simulink model "simulate_filter"  (R2023a)
settings: Solver=VariableStepAuto  StartTime=0.0  StopTime=50  RelTol=1e-3
settings Model: Creator=belov  LastModifiedBy=belov

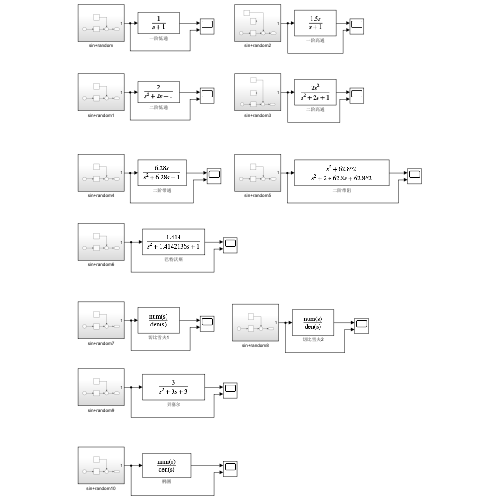
[thumbnail: Simulink's stored preview of the top-level diagram]
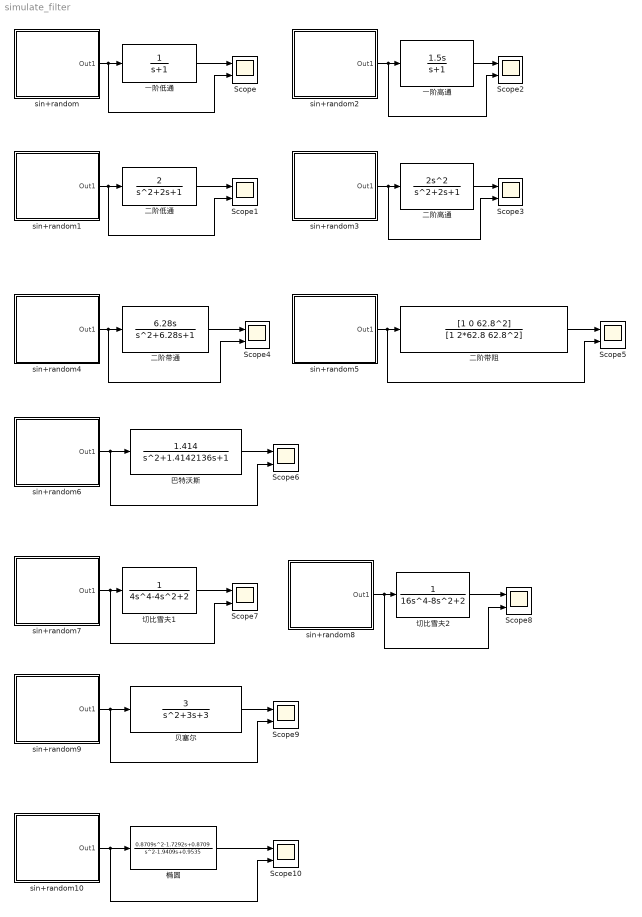
== system simulate_filter ==
  Scope{,1..10} (11 alike) : Scope  NumInputPorts=2
  sin+random : Subsystem
  sin+random1 : Subsystem
  sin+random10 : Subsystem
  sin+random2 : Subsystem
  sin+random3 : Subsystem
  sin+random4 : Subsystem
  sin+random5 : Subsystem
  sin+random6 : Subsystem
  sin+random7 : Subsystem
  sin+random8 : Subsystem
  sin+random9 : Subsystem
  一阶低通 : TransferFcn  Numerator=1  Denominator=[1 1]
  一阶高通 : TransferFcn  Numerator=[1.5 0]  Denominator=[1 1]
  二阶低通 : TransferFcn  Numerator=2
  二阶带通 : TransferFcn  Numerator=[0 6.28 0]  Denominator=[1 6.28 1]
  二阶带阻 : TransferFcn  Numerator=[1 0 62.8^2]  Denominator=[1 2*62.8 62.8^2]
  二阶高通 : TransferFcn  Numerator=[2 0 0]
  切比雪夫1 : TransferFcn  Numerator=1  Denominator=[4 0 -4 0 2]
  切比雪夫2 : TransferFcn  Numerator=1  Denominator=[16 0 -8 0 2]
  巴特沃斯 : TransferFcn  Numerator=[0 0 1.414]  Denominator=[1 1.4142136 1]
  椭圆 : TransferFcn  Numerator="[0.8709   -1.7292    0.8709]"  Denominator="[1.0000   -1.9409    0.9535]"
  贝塞尔 : TransferFcn  Numerator=[3]  Denominator=[1 3 3]
  wires:
  一阶低通/1 -> Scope/1
  sin+random/1(Out1) -> Scope/2, 一阶低通/1
  sin+random1/1(Out1) -> Scope1/2, 二阶低通/1
  二阶低通/1 -> Scope1/1
  sin+random2/1(Out1) -> Scope2/2, 一阶高通/1
  一阶高通/1 -> Scope2/1
  sin+random3/1(Out1) -> Scope3/2, 二阶高通/1
  二阶高通/1 -> Scope3/1
  二阶带通/1 -> Scope4/1
  sin+random4/1(Out1) -> Scope4/2, 二阶带通/1
  sin+random5/1(Out1) -> Scope5/2, 二阶带阻/1
  二阶带阻/1 -> Scope5/1
  sin+random6/1(Out1) -> Scope6/2, 巴特沃斯/1
  巴特沃斯/1 -> Scope6/1
  切比雪夫1/1 -> Scope7/1
  sin+random7/1(Out1) -> 切比雪夫1/1, Scope7/2
  sin+random8/1(Out1) -> Scope8/2, 切比雪夫2/1
  切比雪夫2/1 -> Scope8/1
  sin+random9/1(Out1) -> Scope9/2, 贝塞尔/1
  贝塞尔/1 -> Scope9/1
  sin+random10/1(Out1) -> Scope10/2, 椭圆/1
  椭圆/1 -> Scope10/1

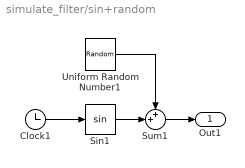
== system simulate_filter/sin+random ==
  Clock1 : Clock
  Sin1 : Trigonometry
  Sum1 : Sum  Inputs=++|
  Uniform Random Number1 : UniformRandomNumber  Minimum=-0.05  Maximum=0.05  SampleTime=0.1
  Out1 : Outport
  wires:
  Sin1/1 -> Sum1/2
  Uniform Random Number1/1 -> Sum1/1
  Clock1/1 -> Sin1/1
  Sum1/1 -> Out1/1

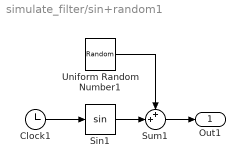
== system simulate_filter/sin+random1 ==
  Clock1 : Clock
  Sin1 : Trigonometry
  Sum1 : Sum  Inputs=++|
  Uniform Random Number1 : UniformRandomNumber  Minimum=-0.05  Maximum=0.05  SampleTime=0.1
  Out1 : Outport
  wires:
  Sum1/1 -> Out1/1
  Clock1/1 -> Sin1/1
  Uniform Random Number1/1 -> Sum1/1
  Sin1/1 -> Sum1/2

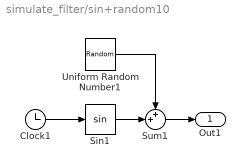
== system simulate_filter/sin+random10 ==
  Clock1 : Clock
  Sin1 : Trigonometry
  Sum1 : Sum  Inputs=++|
  Uniform Random Number1 : UniformRandomNumber  Minimum=-0.1  Maximum=0.1  SampleTime=0.1
  Out1 : Outport
  wires:
  Sin1/1 -> Sum1/2
  Uniform Random Number1/1 -> Sum1/1
  Clock1/1 -> Sin1/1
  Sum1/1 -> Out1/1

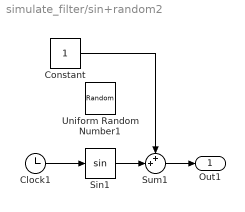
== system simulate_filter/sin+random2 ==
  Clock1 : Clock
  Constant : Constant
  Sin1 : Trigonometry
  Sum1 : Sum  Inputs=++|
  Uniform Random Number1 : UniformRandomNumber  Minimum=-0.1  Maximum=0.1  SampleTime=5
  Out1 : Outport
  wires:
  Sin1/1 -> Sum1/2
  Clock1/1 -> Sin1/1
  Sum1/1 -> Out1/1
  Constant/1 -> Sum1/1

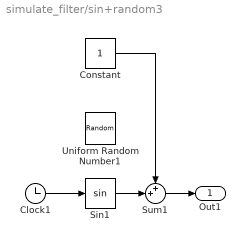
== system simulate_filter/sin+random3 ==
  Clock1 : Clock
  Constant : Constant
  Sin1 : Trigonometry
  Sum1 : Sum  Inputs=++|
  Uniform Random Number1 : UniformRandomNumber  Minimum=-0.1  Maximum=0.1  SampleTime=5
  Out1 : Outport
  wires:
  Sum1/1 -> Out1/1
  Clock1/1 -> Sin1/1
  Sin1/1 -> Sum1/2
  Constant/1 -> Sum1/1

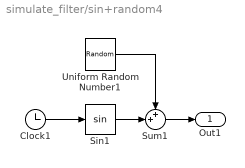
== system simulate_filter/sin+random4 ==
  Clock1 : Clock
  Sin1 : Trigonometry
  Sum1 : Sum  Inputs=++|
  Uniform Random Number1 : UniformRandomNumber  Minimum=-0.05  Maximum=0.05  SampleTime=0.1
  Out1 : Outport
  wires:
  Sum1/1 -> Out1/1
  Clock1/1 -> Sin1/1
  Uniform Random Number1/1 -> Sum1/1
  Sin1/1 -> Sum1/2

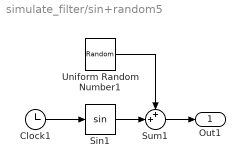
== system simulate_filter/sin+random5 ==
  Clock1 : Clock
  Sin1 : Trigonometry
  Sum1 : Sum  Inputs=++|
  Uniform Random Number1 : UniformRandomNumber  Minimum=-0.05  Maximum=0.05  SampleTime=0.1
  Out1 : Outport
  wires:
  Sin1/1 -> Sum1/2
  Uniform Random Number1/1 -> Sum1/1
  Clock1/1 -> Sin1/1
  Sum1/1 -> Out1/1

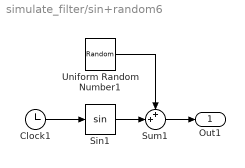
== system simulate_filter/sin+random6 ==
  Clock1 : Clock
  Sin1 : Trigonometry
  Sum1 : Sum  Inputs=++|
  Uniform Random Number1 : UniformRandomNumber  Minimum=-0.1  Maximum=0.1  SampleTime=0.1
  Out1 : Outport
  wires:
  Sin1/1 -> Sum1/2
  Uniform Random Number1/1 -> Sum1/1
  Clock1/1 -> Sin1/1
  Sum1/1 -> Out1/1

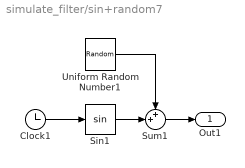
== system simulate_filter/sin+random7 ==
  Clock1 : Clock
  Sin1 : Trigonometry
  Sum1 : Sum  Inputs=++|
  Uniform Random Number1 : UniformRandomNumber  Minimum=-0.1  Maximum=0.1  SampleTime=0.1
  Out1 : Outport
  wires:
  Sum1/1 -> Out1/1
  Clock1/1 -> Sin1/1
  Uniform Random Number1/1 -> Sum1/1
  Sin1/1 -> Sum1/2

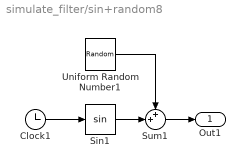
== system simulate_filter/sin+random8 ==
  Clock1 : Clock
  Sin1 : Trigonometry
  Sum1 : Sum  Inputs=++|
  Uniform Random Number1 : UniformRandomNumber  Minimum=-0.1  Maximum=0.1  SampleTime=0.1
  Out1 : Outport
  wires:
  Sin1/1 -> Sum1/2
  Uniform Random Number1/1 -> Sum1/1
  Clock1/1 -> Sin1/1
  Sum1/1 -> Out1/1

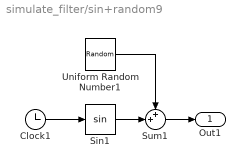
== system simulate_filter/sin+random9 ==
  Clock1 : Clock
  Sin1 : Trigonometry
  Sum1 : Sum  Inputs=++|
  Uniform Random Number1 : UniformRandomNumber  Minimum=-0.1  Maximum=0.1  SampleTime=0.1
  Out1 : Outport
  wires:
  Sin1/1 -> Sum1/2
  Uniform Random Number1/1 -> Sum1/1
  Clock1/1 -> Sin1/1
  Sum1/1 -> Out1/1
